simulink model "Battery_model_M2022b"  (R2024b)
settings: Solver=FixedStepAuto  StartTime=0.0  StopTime=6000  FixedStep=1  RelTol=1e-3
values from neighbouring files (symbols this model uses):
  AH = 2    [Practice_08_MCMC.m]
  etaDischarge = 0.9    [Practice_08_MCMC.m]
  etaR0 = 1.1    [Practice_08_MCMC.m]
  etaV1 = 0.9    [Practice_08_MCMC.m]
  R0 = 0.15    [Practice_08_MCMC.m]
  V1 = 3.3    [Practice_08_MCMC.m]
libraries: nesl_utility x6, fl_lib x4, batteryecm_lib x1
settings Model: SimulationMode=accelerator  Creator=Dario  LastModifiedBy=Lorenzo
settings DebuggingCC: UnconnectedInputMsg=warning  UnconnectedOutputMsg=warning  UnconnectedLineMsg=warning
settings ModelReferenceCC: EnableRefExpFcnMdlSchedulingChecks=on
settings RTWCC: GPUComputeCapability=3.5  DLArmComputeVersion=19.05

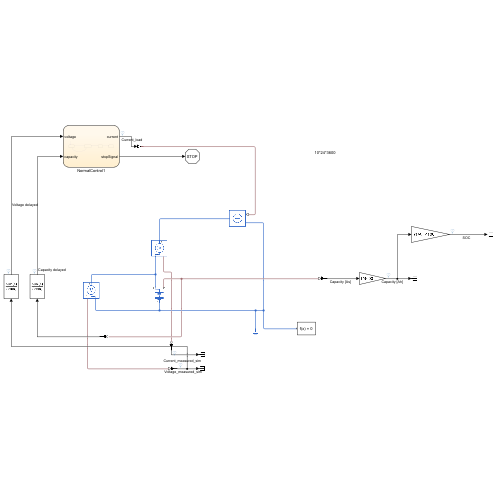
[thumbnail: Simulink's stored preview of the top-level diagram]
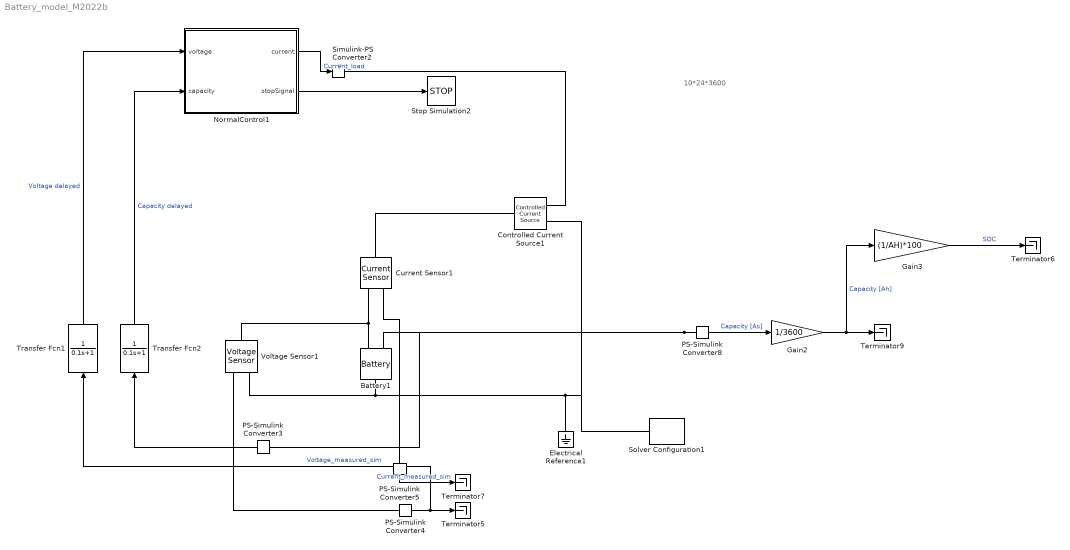
== system Battery_model_M2022b ==
  note: 10*24*3600
  Battery1 : batteryecm_lib/Battery  Vnom=Vnom V  prm_dir=1  R1_dis=2 Ohm  R1_ch=2 Ohm  R1=R0 Ohm  prm_AH=2  AH=AH A*hr  V1=V1 V  AH1=AH1 A*hr  prm_R2=1  R2=2000 Ohm  Tmeas=298.15 K  charge_measurement_port=simscape.enum.battery.enable.yes  prm_dyn=2  Rp1=R1 Ohm  tau1=T1 s  Rp2=R2 Ohm  tau2=T2 s  Rp3=0.005 Ohm  tau3=30 s  Rp4=0.005 Ohm  tau4=30 s  Rp5=0.005 Ohm  tau5=30 s  prm_fade=2  N_fade=100  AH_fade=AH*etaDischarge A*hr  R1_fade=R0*etaR0 Ohm  R1_ch_fade=2.02 Ohm  V1_fade=V1*etaV1 V  prm_age=1  prm_age_OCV=1  OCV_age=0.9  SOC_age=60  Tmeas_age=298.15 K  delta_time_age_vec=[0] d  temperature_age_vec=[273] K  OCV_scaling_age=2.2134e6  OCV_offset_age=1.632e6  temp_exp_age=0.515833569 V  t_exp_age=0.75  Vnom_T2=12 V  R1_T2=2.2 Ohm  R1_T2_dis=2.2 Ohm  R1_T2_ch=2.2 Ohm  V1_T2=11.4 V  R2_T2=2200 Ohm  Rp1_T2=0.005 Ohm  tau1_T2=30 s  Rp2_T2=0.005 Ohm  tau2_T2=30 s  Rp3_T2=0.005 Ohm  tau3_T2=30 s  Rp4_T2=0.005 Ohm  tau4_T2=30 s  Rp5_T2=0.005 Ohm  tau5_T2=30 s  Tmeas2=273.15 K  thermal_port=simscape.enum.thermaleffects.omit  thermal_mass=30000 J/K  i_specify=off  i_priority=None  i=0 A  i_nominal_specify=off  i_nominal_value=1  i_nominal_unit=A  v_specify=off  v_priority=None  v=0 V  v_nominal_specify=off  v_nominal_value=1  v_nominal_unit=V  charge_specify=on  charge_priority=High  charge=0.1 A*hr  charge_nominal_specify=off  charge_nominal_value=1  charge_nominal_unit=A*hr  num_cycles_specify=on  num_cycles_priority=High  num_cycles=N  num_cycles_nominal_specify=off  num_cycles_nominal_value=1  num_cycles_nominal_unit=1  temperature_specify=off  temperature_priority=High  temperature=298.15 K  temperature_nominal_specify=off  temperature_nominal_value=1  temperature_nominal_unit=K
      settings: InternalSimscapePortConfiguration="{\"Bottom\":[],\"Left\":[{\"id\":\"p\",\"label\":\"+\",\"type\":\"foundation.electrical.electrical\"},{\"id\":\"q\",\"label\":\"q\",\"type\":\"output\"}],\"Right\":[{\"id\":\"n\",\"label\":\"-\",\"type\":\"foundation.electrical.electrical\"}],\"Top\":[]}"
  Controlled Current Source1 : fl_lib/Electrical/Electrical Sources/Controlled Current Source
  Current Sensor1 : fl_lib/Electrical/Electrical Sensors/Current Sensor
  Electrical Reference1 : fl_lib/Electrical/Electrical Elements/Electrical Reference
  Gain2 : Gain  Gain=1/3600
  Gain3 : Gain  Gain=(1/AH)*100
  NormalControl1 : Stateflow chart  TreatAsAtomicUnit=on
  PS-Simulink Converter{3..5,8} (4 alike) : nesl_utility/PS-Simulink Converter  PhysicalDomain=network_engine_domain  SubClassName=ps_output  LeftPortType=input  RightPortType=output  PseudoPeriodic=off  Frequencies=[]  VectorFormat=1-D array  Unit=inherit  AffineConversion=off
  Simulink-PS Converter2 : nesl_utility/Simulink-PS Converter  PhysicalDomain=network_engine_domain  SubClassName=ps_input  LeftPortType=input  RightPortType=output  PseudoPeriodic=off  Frequencies=[]  NoiseDistribution=none  NoiseParameters=[]  Unit=1  AffineConversion=off  FilteringAndDerivatives=provide  SimscapeFilterOrder=1  InputFilterTimeConstant=0.001  UdotUserProvided=0
  Solver Configuration1 : nesl_utility/Solver Configuration  PhysicalDomain=network_engine_domain  SubClassName=solver  LeftPortType=input  RightPortType=generic  Tones=[]  Harmonics=[]  SimulateNoise=off  Profile=off  UseLocalSampling=off  EnableSwitchedLinearOptims=on  FrequencyDomain=off  UseCCode=off  RelTol=0.001  AbsTol=1e-06  MinStep=1e-09  ToWorkspace=off  RevertToSquareIcSolve=off  NumHomotopyIterations=100  PhasorMode=off  PhasorModeNumHarmonics=1  ConsistencySolver=NEWTON_FTOL  IndexReductionMethod=DerivativeReplacement  DoDC=off  ResidualTolerance=1e-09  ConsistencyTolSource=GLOBAL  ConsistencyAbsTol=0.001  ConsistencyRelTol=0.001  ConsistencyTolFactor=0.001  UseLocalSolver=off  LocalSolverChoice=NE_BACKWARD_EULER_ADVANCER  ResolveIndetEquations=on  FunctionEvalNumThread=1  LocalSolverSampleTime=0.001  DoFixedCost=off  MaxNonlinIter=3  MaxModeIter=2  ComputeImpulses=off  ImpulseIterations=2  LinearAlgebra=auto  LinearAlgebraNumThread=0  EquationFormulation=NE_TIME_EF  DelaysMemoryBudget=1024  AutomaticFiltering=on  FilteringTimeConstant=0.001  PartitionStorageMethod=AS_NEEDED  PartitionMemoryBudget=1024  PartitionMethod=ROBUST  MultibodyUseLocalSolver=off  MultibodyLocalSolverChoice=ODE1  MultibodyLocalSolverSampleTime=0.001
  Stop Simulation2 : Stop
  Terminator{5..7,9} (4 alike) : Terminator
  Transfer Fcn1 : TransferFcn  Denominator=[0.1 1]
  Transfer Fcn2 : TransferFcn  Denominator=[0.1 1]
  Voltage Sensor1 : fl_lib/Electrical/Electrical Sensors/Voltage Sensor
  wires:
  PS-Simulink Converter3/1 -> Transfer Fcn2/1
  NormalControl1/2(stopSignal) -> Stop Simulation2/1
  Transfer Fcn2/1 -> NormalControl1/2(capacity)  "Capacity delayed"
  NormalControl1/1(current) -> Simulink-PS Converter2/1  "Current_load"
  PS-Simulink Converter8/1 -> Gain2/1  "Capacity [As]"
  Gain2/1 -> Gain3/1, Terminator9/1  "Capacity [Ah]"
  PS-Simulink Converter4/1 -> Terminator5/1, Transfer Fcn1/1  "Voltage_measured_sim"
  Gain3/1 -> Terminator6/1  "SOC"
  PS-Simulink Converter5/1 -> Terminator7/1  "Current_measured_sim"
  Transfer Fcn1/1 -> NormalControl1/1(voltage)  "Voltage delayed"
  connections:
  Current Sensor1/RConn2 -- Voltage Sensor1/LConn1 -- Battery1/LConn1
  Battery1/RConn1 -- Voltage Sensor1/RConn2 -- Solver Configuration1/RConn1 -- Controlled Current Source1/RConn2 -- Electrical Reference1/LConn1
  PS-Simulink Converter8/LConn1 -- Battery1/LConn2 -- PS-Simulink Converter3/LConn1
  PS-Simulink Converter4/LConn1 -- Voltage Sensor1/RConn1
  Current Sensor1/RConn1 -- PS-Simulink Converter5/LConn1
  Controlled Current Source1/RConn1 -- Simulink-PS Converter2/RConn1
  Controlled Current Source1/LConn1 -- Current Sensor1/LConn1

== stateflow chart Battery_model_M2022b/NormalControl1 ==
  state ConstantCurrentDischarge
    entry:
    current = -2;
    exit:
    Ncycles = Ncycles + 1;
  state NoCurrent
    entry:
    current = 0;
  state StopSimulation
    stopSignal = 1;
  state ConstantCurrentCharge
    entry:
    current = 2;
  (default) -> ConstantCurrentCharge : {Ncycles = 0;
      | stopSignal = 0;}
  ConstantCurrentDischarge -> NoCurrent [order 2] : [voltage<2.7]
  NoCurrent -> StopSimulation : after(600, sec)
  ConstantCurrentCharge -> ConstantCurrentDischarge : [capacity/3600 > 1.75]
  ConstantCurrentDischarge -> ConstantCurrentCharge [order 1] : [voltage < 2.7 && Ncycles < 50]
  data: voltage input; current output; Ncycles local; capacity input; stopSignal output =0
